simulink model "Bandwidth_demo"  (R2022b)
settings: Solver=VariableStepAuto  StartTime=0.0  StopTime=Inf  RelTol=1e-3
libraries: aerolibanimutils x1
settings Model: Creator=fades  LastModifiedBy=fades

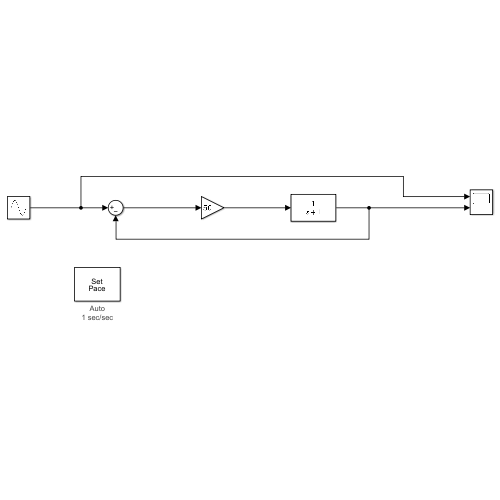
[thumbnail: Simulink's stored preview of the top-level diagram]
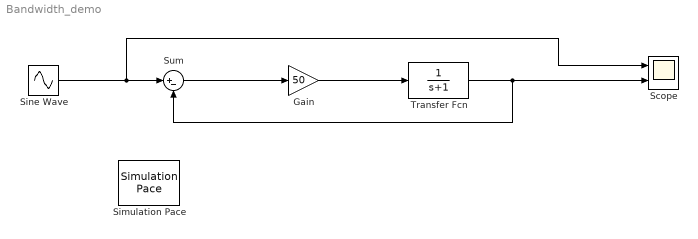
== system Bandwidth_demo ==
  Gain : Gain  Gain=50
  Scope : Scope  NumInputPorts=2
  Simulation Pace : aerolibanimutils/Simulation Pace  SimulationPace=1  SleepMode=Auto  OutputPaceError=off  SampleTime=1/30
  Sine Wave : Sin  Frequency=1000  SampleTime=0
  Sum : Sum  Inputs=|+-
  Transfer Fcn : TransferFcn  Denominator=[1 1]
  wires:
  Sine Wave/1 -> Scope/1, Sum/1
  Sum/1 -> Gain/1
  Gain/1 -> Transfer Fcn/1
  Transfer Fcn/1 -> Sum/2, Scope/2
